simulink model "MotorController"  (R2022a)
settings: Solver=VariableStepAuto  StartTime=0.0  StopTime=10.0  RelTol=1e-3
settings Model: Creator=The MathWorks, Inc.  LastModifiedBy=The MathWorks, Inc.
settings SolverCC: MaxZcPerStep=1
settings DebuggingCC: UnconnectedInputMsg=warning  UnconnectedOutputMsg=warning  UnconnectedLineMsg=warning
settings RTWCC: DLArmComputeVersion=19.05

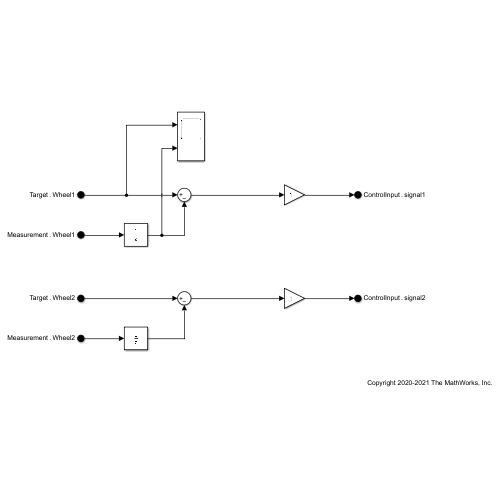
[thumbnail: Simulink's stored preview of the top-level diagram]
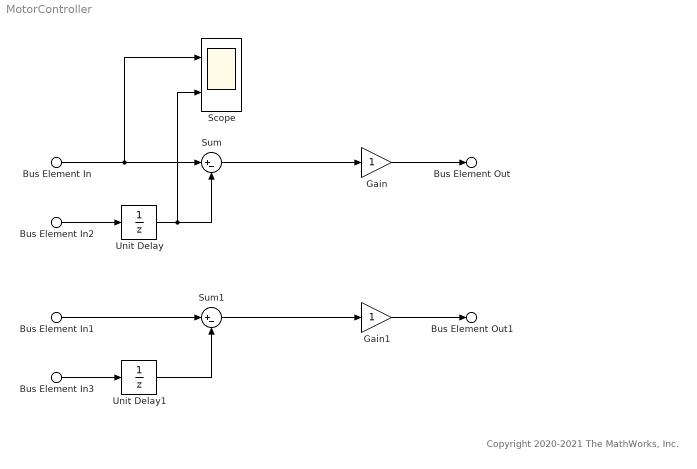
== system MotorController ==
  note: Copyright 2020-2021 The MathWorks, Inc.
  Bus Element In1 : Inport  PortName=Target  Element=Wheel2
  Bus Element In : Inport  PortName=Target  Element=Wheel1
  Bus Element In3 : Inport  Port=2  PortName=Measurement  Element=Wheel2
  Bus Element In2 : Inport  Port=2  PortName=Measurement  Element=Wheel1
  Gain : Gain
  Gain1 : Gain
  Scope : Scope  NumInputPorts=2
  Sum : Sum  Inputs=|+-
  Sum1 : Sum  Inputs=|+-
  Unit Delay : UnitDelay  SampleTime=-1  HasFrameUpgradeWarning=on
  Unit Delay1 : UnitDelay  SampleTime=-1  HasFrameUpgradeWarning=on
  Bus Element Out : Outport  PortName=ControlInput  Element=signal1
  Bus Element Out1 : Outport  PortName=ControlInput  Element=signal2
  wires:
  Bus Element In/1 -> Scope/1, Sum/1
  Bus Element In2/1 -> Unit Delay/1
  Bus Element In1/1 -> Sum1/1
  Bus Element In3/1 -> Unit Delay1/1
  Sum/1 -> Gain/1
  Sum1/1 -> Gain1/1
  Gain/1 -> Bus Element Out/1
  Gain1/1 -> Bus Element Out1/1
  Unit Delay/1 -> Scope/2, Sum/2
  Unit Delay1/1 -> Sum1/2
